simulink model "test"  (R2021a)
settings: Solver=VariableStepAuto  StartTime=0.0  StopTime=10.0  RelTol=1e-3
settings Model: Creator=fedeoli  LastModifiedBy=FusionLab
settings SolverCC: AlgebraicLoopSolver=TrustRegion
settings DebuggingCC: SFMachineParentedDataDiag=warning

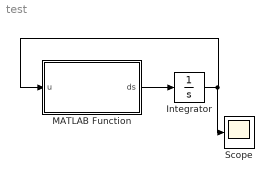
== system test ==
  Integrator : Integrator
  MATLAB Function : MATLAB Function  TreatAsAtomicUnit=on
  Scope : Scope
  wires:
  MATLAB Function/1(ds) -> Integrator/1
  Integrator/1 -> Scope/1, MATLAB Function/1(u)

== matlab function test/MATLAB Function ==
  data: u input; ds output; params parameter
function ds = fcn(u,params)
    ds = params.m*u + params.I(3,3);
end
